simulink model "Current_Fed_DC_DC_Converter_Code_Equivalent_v4"  (R2020a)
settings: Solver=ode3  StartTime=0.0  StopTime=0.4  MaxStep=1e-5  MinStep=1e-7  RelTol=1e-6
InitFcn:
  | %Supply
  | V_supply = 415;
  | f_supply = 50;
  | 
  | %DC_Bus
  | C_filt = 220e-6
  | L_dc = 100e-6;
  | C_out = 560e-3;
  | 
  | %Transformer
  | P_TX = 10e3;
  | V_pri = 36;
  | V_sec = 1;
  | L_leak = 0;
  | R_leak = 0;
  | L_mag = inf;
  | R_mag = inf;
  | 
  | %Control
  | f_sw = 15e3;
  | tss_conv = 0.1;
  | V_ref = 1480;
  | Kp_V = 1;
  | Ki_V = 0.001;
  | I_ref = 2920;
  | Kp_I = 0.025;
  | Ki_I = 0.000001;
  | PS_max = 180;
  | Carr_offset = 1;
  | Carr_scale = 0.5;
  | Duty_scale = 0.01;
  | Duty_fix = 50;
  | Duty_max = 75;
  | Duty_min = 0;
  | f_chop = 1e3;
  | Duty_chop = 40;
  | 
  | %Harmonic_Correction
  | P_inj = 50;
  | f_inj = 50;
  | L_inj = 10e-6;
  | R_inj = 1;
  | Vpri_inj = 1;
  | Vsec_inj = 70;
  | Rleak_inj = 1e-3;
  | Lleak_inj = 12e-6;
  | R_inj = 0.1;
  | Rmag_inj = 1e-3;
  | Lmag_inj = 1e-3;
  | 
  | %Sensor
  | ADC_Res = 4096;
  | I_sense = 1/700;
  | V_sense = 1/50;
  | 
  | %Faults
  | OV_limit = 18.25;
  | UV_limit = 17.5;
  | OC_limit = 515;
  | UC_limit = 22;
  | 
  | %Load
  | R_load = 0.036;
libraries: powerlib x109, powerlib_meascontrol x30, simulink x5, slctrlblks x2
(part 1 of 3)
settings Model: Creator=Duke  LastModifiedBy=Testinglaptop2
settings DataIOCC: ReturnWorkspaceOutputs=off

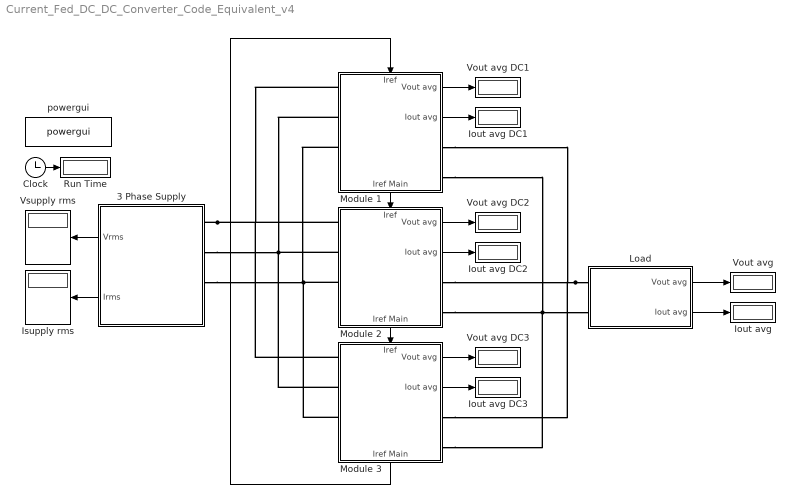
== system Current_Fed_DC_DC_Converter_Code_Equivalent_v4 ==
  3 Phase Supply : Subsystem
      settings: PortSchema="{\"entries\":[{\"content\":{\"sides\":[{\"content\":{\"connectorIds\":[\"Out1\",\"Out2\"]},\"type\":\"ConnectorPlacement.EquallySpacedRectSide\",\"uuid\":\"0ec2aa27-c625-4e75-9974-9a1c04d8f7d1\"},{\"content\":{\"connectorIds\":[\"RConn1\",\"RConn2\",\"RConn3\",\"RConn4\"],\"side\":\"RIGHT\"},\"type\":\"ConnectorPlacement.EquallySpacedRectSide\",\"uuid\":\"47308d37-cd5f-48af-b8fb-0231d0d207f3\"},{\"content\":{\"connectorIds\":[],\"side\":\"TOP\"},\"type\":\"ConnectorPlacement.EquallySpacedRectSide\",\"uuid\":\"36312fad-683d-4b15-bbb8-6a51adddf298\"},{\"content\":{\"connectorIds\":[],\"side\":\"BOTTOM\"},\"type\":\"ConnectorPlacement.EquallySpacedRectSide\",\"uuid\":\"2222870e-1ee8-49e9-8ac2-78ebac8795b0\"}]},\"type\":\"ConnectorPlacement.EquallySpacedConnector\",\"uuid\":\"d2540331-bb7c-4989-bdfb-e9d86418b7e1\"}],\"packageUris\":[\"http://schema.mathworks.com/mf0/Connector/19700101\"],\"version\":\"1.0\"}"
  Clock : Clock
  Iout avg : Display
  Iout avg DC1 : Display
  Iout avg DC2 : Display
  Iout avg DC3 : Display
  Isupply rms : Display
  Load : Subsystem
  Module 1 : Subsystem
      settings: PortSchema="{\"entries\":[{\"content\":{\"sides\":[{\"content\":{\"connectorIds\":[\"LConn1\",\"LConn2\",\"LConn3\",\"LConn4\"]},\"type\":\"ConnectorPlacement.EquallySpacedRectSide\",\"uuid\":\"6cae0e2c-353b-4935-ad30-0e7f8192a6e9\"},{\"content\":{\"connectorIds\":[\"Out1\",\"Out2\",\"RConn1\",\"RConn2\"],\"side\":\"RIGHT\"},\"type\":\"ConnectorPlacement.EquallySpacedRectSide\",\"uuid\":\"f189d0b5-f9e6-4211-8a45-ed2746b7bcfd\"},{\"content\":{\"connectorIds\":[\"In1\"],\"side\":\"TOP\"},\"type\":\"ConnectorPlacement.EquallySpacedRectSide\",\"uuid\":\"18788e66-a885-4273-91b7-13b54a877d5d\"},{\"content\":{\"connectorIds\":[\"Out3\"],\"side\":\"BOTTOM\"},\"type\":\"ConnectorPlacement.EquallySpacedRectSide\",\"uuid\":\"bb6cd510-79be-413f-a402-cf5e288de2de\"}]},\"type\":\"ConnectorPlacement.EquallySpacedConnector\",\"uuid\":\"96fd3dee-bad9-4110-8bef-6c3594df368f\"}],\"packageUris\":[\"http://schema.mathworks.com/mf0/Connector/19700101\"],\"version\":\"1.0\"}"
  Module 2 : Subsystem
      settings: PortSchema="{\"entries\":[{\"content\":{\"sides\":[{\"content\":{\"connectorIds\":[\"LConn1\",\"LConn2\",\"LConn3\",\"LConn4\"]},\"type\":\"ConnectorPlacement.EquallySpacedRectSide\",\"uuid\":\"6cae0e2c-353b-4935-ad30-0e7f8192a6e9\"},{\"content\":{\"connectorIds\":[\"Out1\",\"Out2\",\"RConn1\",\"RConn2\"],\"side\":\"RIGHT\"},\"type\":\"ConnectorPlacement.EquallySpacedRectSide\",\"uuid\":\"f189d0b5-f9e6-4211-8a45-ed2746b7bcfd\"},{\"content\":{\"connectorIds\":[\"In1\"],\"side\":\"TOP\"},\"type\":\"ConnectorPlacement.EquallySpacedRectSide\",\"uuid\":\"18788e66-a885-4273-91b7-13b54a877d5d\"},{\"content\":{\"connectorIds\":[\"Out3\"],\"side\":\"BOTTOM\"},\"type\":\"ConnectorPlacement.EquallySpacedRectSide\",\"uuid\":\"bb6cd510-79be-413f-a402-cf5e288de2de\"}]},\"type\":\"ConnectorPlacement.EquallySpacedConnector\",\"uuid\":\"96fd3dee-bad9-4110-8bef-6c3594df368f\"}],\"packageUris\":[\"http://schema.mathworks.com/mf0/Connector/19700101\"],\"version\":\"1.0\"}"
  Module 3 : Subsystem
      settings: PortSchema="{\"entries\":[{\"content\":{\"sides\":[{\"content\":{\"connectorIds\":[\"LConn1\",\"LConn2\",\"LConn3\",\"LConn4\"]},\"type\":\"ConnectorPlacement.EquallySpacedRectSide\",\"uuid\":\"6cae0e2c-353b-4935-ad30-0e7f8192a6e9\"},{\"content\":{\"connectorIds\":[\"Out1\",\"Out2\",\"RConn1\",\"RConn2\"],\"side\":\"RIGHT\"},\"type\":\"ConnectorPlacement.EquallySpacedRectSide\",\"uuid\":\"f189d0b5-f9e6-4211-8a45-ed2746b7bcfd\"},{\"content\":{\"connectorIds\":[\"In1\"],\"side\":\"TOP\"},\"type\":\"ConnectorPlacement.EquallySpacedRectSide\",\"uuid\":\"18788e66-a885-4273-91b7-13b54a877d5d\"},{\"content\":{\"connectorIds\":[\"Out3\"],\"side\":\"BOTTOM\"},\"type\":\"ConnectorPlacement.EquallySpacedRectSide\",\"uuid\":\"bb6cd510-79be-413f-a402-cf5e288de2de\"}]},\"type\":\"ConnectorPlacement.EquallySpacedConnector\",\"uuid\":\"96fd3dee-bad9-4110-8bef-6c3594df368f\"}],\"packageUris\":[\"http://schema.mathworks.com/mf0/Connector/19700101\"],\"version\":\"1.0\"}"
  Run Time : Display
  Vout avg : Display
  Vout avg DC1 : Display
  Vout avg DC2 : Display
  Vout avg DC3 : Display
  Vsupply rms : Display
  powergui : powerlib/powergui  Priority=1  SimulationMode=Discrete  SampleTime=1e-6  frequency=60  Iterations=50  frequencyindice=0  Pbase=100e6  ErrMax=1e-4  UnitsV=kV  UnitsW=MW  buscounter=0  FunctionMessages=off  echomessages=off  EnableUseOfTLC=off  CurrentSourceSwitches=off  DisableSnubberDevices=off  DisableRonSwitches=off  DisableVfSwitches=off  DisplayEquations=off  AutomaticDiscreteSolvers=off  SolverType=Tustin/Backward Euler (TBE)  Interpol=off  ExternalGateDelay=off  methode=off  Ts=100  x0status=blocks  SPID=on  SwTol=0  HookPort=off  NonlinearTolerance=1e-4  nMaxIteration=100  ContinueOnMaxIteration=off  RestoreLinks=warning  ResistiveCurrentMeasurement=off  Frange=[0:2:500]  Ylog=off  Xlog=on  ShowGrid=off  save=off  variable=ZData  structure=Supply  ZoomFFT=off  StartTime=0.1  cycles=5  DisplayStyle=1  fundamental=50  FreqAxis=off  MaxFrequency=1000  frequencyindicesteady=1  RmsSteady=1  display=off
  wires:
  Clock/1 -> Run Time/1
  Load/2(Iout avg) -> Iout avg/1
  Load/1(Vout avg) -> Vout avg/1
  Module 1/1(Vout avg) -> Vout avg DC1/1
  Module 1/2(Iout avg) -> Iout avg DC1/1
  3 Phase Supply/2(Irms) -> Isupply rms/1
  3 Phase Supply/1(Vrms) -> Vsupply rms/1
  Module 2/2(Iout avg) -> Iout avg DC2/1
  Module 2/1(Vout avg) -> Vout avg DC2/1
  Module 1/3(Iref Main) -> Module 2/1(Iref)
  Module 2/3(Iref Main) -> Module 3/1(Iref)
  Module 3/3(Iref Main) -> Module 1/1(Iref)
  Module 3/1(Vout avg) -> Vout avg DC3/1
  Module 3/2(Iout avg) -> Iout avg DC3/1
  connections:
  3 Phase Supply/RConn1 -- Module 3/LConn1 -- Module 1/LConn1 -- Module 2/LConn1
  Module 1/LConn3 -- 3 Phase Supply/RConn3 -- Module 3/LConn3 -- Module 2/LConn3
  Module 2/RConn2 -- Load/LConn2 -- Module 3/RConn2 -- Module 1/RConn2
  Load/LConn1 -- Module 3/RConn1 -- Module 1/RConn1 -- Module 2/RConn1
  3 Phase Supply/RConn2 -- Module 3/LConn2 -- Module 1/LConn2 -- Module 2/LConn2

== system Current_Fed_DC_DC_Converter_Code_Equivalent_v4/3 Phase Supply ==
  3 Phase Source : powerlib/Electrical Sources/Three-Phase Programmable Voltage Source  PositiveSequence="[V_supply  0 f_supply]"  VariationEntity=None  VariationType=Table of time-amplitude pairs  VariationTypeAlt=Step  VariationStep=0.5  VariationRate=10  VariationMagnitude=0.3  VariationFrequency=2  VariationTiming=[1 2]  VariationPhaseA=off  Amplitudes=[1 0.8 1.2 1.0]  TimeValues=[0 0.1 0.15 0.2]  HarmonicGeneration=off  HarmonicA=[3 0.2 -25 0]  HarmonicB=[2 0.15 35 2]  Timing="[0.05  3]"  BusType=swing  Pref=0  Qref=0  Qmin=-inf  Qmax=inf
  Measurement Input : Subsystem
      settings: PortSchema="{\"entries\":[{\"content\":{\"sides\":[{\"content\":{\"connectorIds\":[\"LConn1\",\"LConn2\",\"LConn3\"]},\"type\":\"ConnectorPlacement.EquallySpacedRectSide\",\"uuid\":\"3be9e5d9-1b35-404b-9f43-9e3a478b191c\"},{\"content\":{\"connectorIds\":[\"RConn1\",\"RConn2\",\"RConn3\"],\"side\":\"RIGHT\"},\"type\":\"ConnectorPlacement.EquallySpacedRectSide\",\"uuid\":\"eba31e05-cbe5-4e3c-a514-94f682603724\"},{\"content\":{\"connectorIds\":[],\"side\":\"TOP\"},\"type\":\"ConnectorPlacement.EquallySpacedRectSide\",\"uuid\":\"b07c13d9-dc8e-463c-8536-a0457c056d42\"},{\"content\":{\"connectorIds\":[\"Out1\",\"Out2\"],\"side\":\"BOTTOM\"},\"type\":\"ConnectorPlacement.EquallySpacedRectSide\",\"uuid\":\"1df26e5f-c204-4844-b869-5c4c651719e7\"}]},\"type\":\"ConnectorPlacement.EquallySpacedConnector\",\"uuid\":\"ca8d1314-165f-4aba-a39c-e8b968dfc3e9\"}],\"packageUris\":[\"http://schema.mathworks.com/mf0/Connector/19700101\"],\"version\":\"1.0\"}"
  Rphase : PMIOPort  Side=Right
  Yphase : PMIOPort  Port=2  Side=Right
  Bphase : PMIOPort  Port=3  Side=Right
  Neutral : PMIOPort  Port=4  Side=Right
  Vrms : Outport
  Irms : Outport  Port=2
  wires:
  Measurement Input/2(Vrms) -> Vrms/1
  Measurement Input/1(Irms) -> Irms/1
  connections:
  Measurement Input/RConn1 -- Rphase/RConn1
  Measurement Input/RConn2 -- Yphase/RConn1
  3 Phase Source/LConn1 -- Neutral/RConn1
  Measurement Input/RConn3 -- Bphase/RConn1
  3 Phase Source/RConn2 -- Measurement Input/LConn2
  3 Phase Source/RConn1 -- Measurement Input/LConn1
  3 Phase Source/RConn3 -- Measurement Input/LConn3

== system Current_Fed_DC_DC_Converter_Code_Equivalent_v4/Load ==
  Io avg : powerlib_meascontrol/Measurements/Mean  Freq=f_supply  Vinit=0  Ts=0
  Iout : powerlib/Measurements/Current Measurement  PhasorSimulation=off  OutputType=Complex  PSBequivalent=0
  Load 1 : powerlib/Elements/Series RLC Branch  LConnTagsString=__new0  RConnTagsString=__new0  BranchType=R  Resistance=R_load  Inductance=1e-3  SetiL0=off  InitialCurrent=0  Capacitance=1e-6  Setx0=off  InitialVoltage=0  Measurements=None
  Load 2 : powerlib/Elements/Series RLC Branch  LConnTagsString=__new0  RConnTagsString=__new0  BranchType=R  Resistance=R_load  Inductance=1e-3  SetiL0=off  InitialCurrent=0  Capacitance=1e-6  Setx0=off  InitialVoltage=0  Measurements=None
  Load 3 : powerlib/Elements/Series RLC Branch  LConnTagsString=__new0  RConnTagsString=__new0  BranchType=R  Resistance=R_load  Inductance=1e-3  SetiL0=off  InitialCurrent=0  Capacitance=1e-6  Setx0=off  InitialVoltage=0  Measurements=None
  Output Parameters : Scope  NumInputPorts=2
  Vo avg : powerlib_meascontrol/Measurements/Mean  Freq=f_supply  Vinit=0  Ts=0
  Vout : powerlib/Measurements/Voltage Measurement  PhasorSimulation=off  OutputType=Complex  PSBequivalent=0
  +ve : PMIOPort  Side=Left
  -ve : PMIOPort  Port=2  Side=Left
  Vout avg : Outport
  Iout avg : Outport  Port=2
  wires:
  Io avg/1 -> Iout avg/1  "Io avg"
  Vo avg/1 -> Vout avg/1  "Vo avg"
  Iout/1 -> Io avg/1, Output Parameters/1  "Iout"
  Vout/1 -> Vo avg/1, Output Parameters/2  "Vout"
  connections:
  Vout/LConn2 -- -ve/RConn1 -- Load 1/RConn1 -- Load 2/RConn1 -- Load 3/RConn1
  Iout/LConn1 -- +ve/RConn1
  Vout/LConn1 -- Load 2/LConn1 -- Load 1/LConn1 -- Iout/RConn1 -- Load 3/LConn1

== system Current_Fed_DC_DC_Converter_Code_Equivalent_v4/Module 1 ==
  Iref : Inport
  3 Phase Rectifier : Subsystem
  DC DC Converter : Subsystem
      settings: PortSchema="{\"entries\":[{\"content\":{\"sides\":[{\"content\":{\"connectorIds\":[\"LConn1\",\"LConn2\"]},\"type\":\"ConnectorPlacement.EquallySpacedRectSide\",\"uuid\":\"37f51f67-5e78-4255-afaf-84866755c3fb\"},{\"content\":{\"connectorIds\":[\"RConn1\",\"RConn2\"],\"side\":\"RIGHT\"},\"type\":\"ConnectorPlacement.EquallySpacedRectSide\",\"uuid\":\"2b53282d-d294-4b9e-9ae3-da15b818eb82\"},{\"content\":{\"connectorIds\":[\"In1\"],\"side\":\"TOP\"},\"type\":\"ConnectorPlacement.EquallySpacedRectSide\",\"uuid\":\"215168e2-cc4d-42b6-b915-d0598b09a452\"},{\"content\":{\"connectorIds\":[\"Out1\",\"Out2\",\"Out3\"],\"side\":\"BOTTOM\"},\"type\":\"ConnectorPlacement.EquallySpacedRectSide\",\"uuid\":\"f9f369b9-2556-4108-8119-ee65139e69f0\"}]},\"type\":\"ConnectorPlacement.EquallySpacedConnector\",\"uuid\":\"d8162db6-aadc-4169-8971-befd1c7fce06\"}],\"packageUris\":[\"http://schema.mathworks.com/mf0/Connector/19700101\"],\"version\":\"1.0\"}"
  Rphase : PMIOPort  Side=Left
  Yphase : PMIOPort  Port=2  Side=Left
  Bphase : PMIOPort  Port=3  Side=Left
  +ve OUT : PMIOPort  Port=4  Side=Right
  -ve OUT : PMIOPort  Port=5  Side=Right
  Neutral : PMIOPort  Port=6  Side=Left
  Vout avg : Outport
  Iout avg : Outport  Port=2
  Iref Main : Outport  Port=3
  wires:
  DC DC Converter/3(Vdc avg) -> Vout avg/1
  DC DC Converter/2(Idc avg) -> Iout avg/1
  DC DC Converter/1(Iref Main) -> Iref Main/1
  Iref/1 -> DC DC Converter/1(Iref)
  connections:
  3 Phase Rectifier/LConn3 -- Bphase/RConn1
  DC DC Converter/LConn1 -- 3 Phase Rectifier/RConn1
  DC DC Converter/LConn2 -- 3 Phase Rectifier/RConn2
  DC DC Converter/RConn2 -- -ve OUT/RConn1
  DC DC Converter/RConn1 -- +ve OUT/RConn1
  3 Phase Rectifier/LConn2 -- Yphase/RConn1
  3 Phase Rectifier/LConn1 -- Rphase/RConn1
  Neutral/RConn1 -- 3 Phase Rectifier/LConn4

== system Current_Fed_DC_DC_Converter_Code_Equivalent_v4/Module 2 ==
  Iref : Inport
  3 Phase Rectifier : Subsystem
  DC DC Converter : Subsystem
      settings: PortSchema="{\"entries\":[{\"content\":{\"sides\":[{\"content\":{\"connectorIds\":[\"LConn1\",\"LConn2\"]},\"type\":\"ConnectorPlacement.EquallySpacedRectSide\",\"uuid\":\"37f51f67-5e78-4255-afaf-84866755c3fb\"},{\"content\":{\"connectorIds\":[\"RConn1\",\"RConn2\"],\"side\":\"RIGHT\"},\"type\":\"ConnectorPlacement.EquallySpacedRectSide\",\"uuid\":\"2b53282d-d294-4b9e-9ae3-da15b818eb82\"},{\"content\":{\"connectorIds\":[\"In1\"],\"side\":\"TOP\"},\"type\":\"ConnectorPlacement.EquallySpacedRectSide\",\"uuid\":\"215168e2-cc4d-42b6-b915-d0598b09a452\"},{\"content\":{\"connectorIds\":[\"Out1\",\"Out2\",\"Out3\"],\"side\":\"BOTTOM\"},\"type\":\"ConnectorPlacement.EquallySpacedRectSide\",\"uuid\":\"f9f369b9-2556-4108-8119-ee65139e69f0\"}]},\"type\":\"ConnectorPlacement.EquallySpacedConnector\",\"uuid\":\"d8162db6-aadc-4169-8971-befd1c7fce06\"}],\"packageUris\":[\"http://schema.mathworks.com/mf0/Connector/19700101\"],\"version\":\"1.0\"}"
  Rphase : PMIOPort  Side=Left
  Yphase : PMIOPort  Port=2  Side=Left
  Bphase : PMIOPort  Port=3  Side=Left
  +ve OUT : PMIOPort  Port=4  Side=Right
  -ve OUT : PMIOPort  Port=5  Side=Right
  Neutral : PMIOPort  Port=6  Side=Left
  Vout avg : Outport
  Iout avg : Outport  Port=2
  Iref Main : Outport  Port=3
  wires:
  Iref/1 -> DC DC Converter/1(Iref)
  DC DC Converter/1(Iref Main) -> Iref Main/1
  DC DC Converter/2(Idc avg) -> Iout avg/1
  DC DC Converter/3(Vdc avg) -> Vout avg/1
  connections:
  Neutral/RConn1 -- 3 Phase Rectifier/LConn4
  3 Phase Rectifier/LConn1 -- Rphase/RConn1
  3 Phase Rectifier/LConn2 -- Yphase/RConn1
  DC DC Converter/RConn1 -- +ve OUT/RConn1
  DC DC Converter/RConn2 -- -ve OUT/RConn1
  DC DC Converter/LConn2 -- 3 Phase Rectifier/RConn2
  DC DC Converter/LConn1 -- 3 Phase Rectifier/RConn1
  3 Phase Rectifier/LConn3 -- Bphase/RConn1

== system Current_Fed_DC_DC_Converter_Code_Equivalent_v4/Module 3 ==
  Iref : Inport
  3 Phase Rectifier : Subsystem
  DC DC Converter : Subsystem
      settings: PortSchema="{\"entries\":[{\"content\":{\"sides\":[{\"content\":{\"connectorIds\":[\"LConn1\",\"LConn2\"]},\"type\":\"ConnectorPlacement.EquallySpacedRectSide\",\"uuid\":\"37f51f67-5e78-4255-afaf-84866755c3fb\"},{\"content\":{\"connectorIds\":[\"RConn1\",\"RConn2\"],\"side\":\"RIGHT\"},\"type\":\"ConnectorPlacement.EquallySpacedRectSide\",\"uuid\":\"2b53282d-d294-4b9e-9ae3-da15b818eb82\"},{\"content\":{\"connectorIds\":[\"In1\"],\"side\":\"TOP\"},\"type\":\"ConnectorPlacement.EquallySpacedRectSide\",\"uuid\":\"215168e2-cc4d-42b6-b915-d0598b09a452\"},{\"content\":{\"connectorIds\":[\"Out1\",\"Out2\",\"Out3\"],\"side\":\"BOTTOM\"},\"type\":\"ConnectorPlacement.EquallySpacedRectSide\",\"uuid\":\"f9f369b9-2556-4108-8119-ee65139e69f0\"}]},\"type\":\"ConnectorPlacement.EquallySpacedConnector\",\"uuid\":\"d8162db6-aadc-4169-8971-befd1c7fce06\"}],\"packageUris\":[\"http://schema.mathworks.com/mf0/Connector/19700101\"],\"version\":\"1.0\"}"
  Rphase : PMIOPort  Side=Left
  Yphase : PMIOPort  Port=2  Side=Left
  Bphase : PMIOPort  Port=3  Side=Left
  +ve OUT : PMIOPort  Port=4  Side=Right
  -ve OUT : PMIOPort  Port=5  Side=Right
  Neutral : PMIOPort  Port=6  Side=Left
  Vout avg : Outport
  Iout avg : Outport  Port=2
  Iref Main : Outport  Port=3
  wires:
  Iref/1 -> DC DC Converter/1(Iref)
  DC DC Converter/1(Iref Main) -> Iref Main/1
  DC DC Converter/2(Idc avg) -> Iout avg/1
  DC DC Converter/3(Vdc avg) -> Vout avg/1
  connections:
  Neutral/RConn1 -- 3 Phase Rectifier/LConn4
  3 Phase Rectifier/LConn1 -- Rphase/RConn1
  3 Phase Rectifier/LConn2 -- Yphase/RConn1
  DC DC Converter/RConn1 -- +ve OUT/RConn1
  DC DC Converter/RConn2 -- -ve OUT/RConn1
  DC DC Converter/LConn2 -- 3 Phase Rectifier/RConn2
  DC DC Converter/LConn1 -- 3 Phase Rectifier/RConn1
  3 Phase Rectifier/LConn3 -- Bphase/RConn1

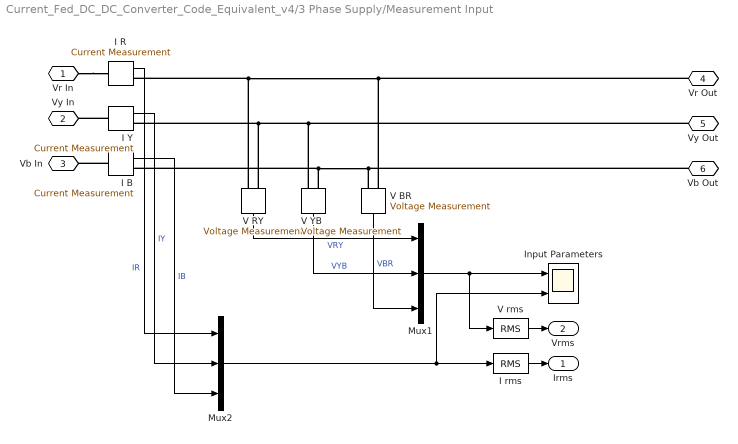
== system Current_Fed_DC_DC_Converter_Code_Equivalent_v4/3 Phase Supply/Measurement Input ==
  I B : powerlib/Measurements/Current Measurement  PhasorSimulation=off  OutputType=Complex  PSBequivalent=0
  I R : powerlib/Measurements/Current Measurement  PhasorSimulation=off  OutputType=Complex  PSBequivalent=0
  I Y : powerlib/Measurements/Current Measurement  PhasorSimulation=off  OutputType=Complex  PSBequivalent=0
  I rms : powerlib_meascontrol/Measurements/RMS  TrueRMS=on  Freq=f_supply  RMSInit=0  Ts=0
  Input Parameters : Scope  NumInputPorts=2
  Mux1 : Mux  Inputs=3
  Mux2 : Mux  Inputs=3
  V BR : powerlib/Measurements/Voltage Measurement  PhasorSimulation=off  OutputType=Complex  PSBequivalent=0
  V RY : powerlib/Measurements/Voltage Measurement  PhasorSimulation=off  OutputType=Complex  PSBequivalent=0
  V YB : powerlib/Measurements/Voltage Measurement  PhasorSimulation=off  OutputType=Complex  PSBequivalent=0
  V rms : powerlib_meascontrol/Measurements/RMS  TrueRMS=on  Freq=f_supply  RMSInit=0  Ts=0
  Vr In : PMIOPort  Side=Left
  Vy In : PMIOPort  Port=2  Side=Left
  Vb In : PMIOPort  Port=3  Side=Left
  Vr Out : PMIOPort  Port=4  Side=Right
  Vy Out : PMIOPort  Port=5  Side=Right
  Vb Out : PMIOPort  Port=6  Side=Right
  Irms : Outport
  Vrms : Outport  Port=2
  wires:
  Mux2/1 -> Input Parameters/2, I rms/1
  V RY/1 -> Mux1/1  "VRY"
  Mux1/1 -> Input Parameters/1, V rms/1
  I B/1 -> Mux2/3  "IB"
  I Y/1 -> Mux2/2  "IY"
  I R/1 -> Mux2/1  "IR"
  V BR/1 -> Mux1/3  "VBR"
  V YB/1 -> Mux1/2  "VYB"
  I rms/1 -> Irms/1
  V rms/1 -> Vrms/1
  connections:
  V YB/LConn2 -- I B/RConn1 -- Vb Out/RConn1 -- V BR/LConn1
  V RY/LConn1 -- Vr Out/RConn1 -- V BR/LConn2 -- I R/RConn1
  Vr In/RConn1 -- I R/LConn1
  V RY/LConn2 -- Vy Out/RConn1 -- V YB/LConn1 -- I Y/RConn1
  I B/LConn1 -- Vb In/RConn1
  I Y/LConn1 -- Vy In/RConn1

== system Current_Fed_DC_DC_Converter_Code_Equivalent_v4/Module 1/3 Phase Rectifier ==
  3 Phase Rectifier : Subsystem
  Filter : Subsystem
  Rphase : PMIOPort  Side=Left
  Yphase : PMIOPort  Port=2  Side=Left
  Bphase : PMIOPort  Port=3  Side=Left
  +ve : PMIOPort  Port=4  Side=Right
  -ve : PMIOPort  Port=5  Side=Right
  Neutral : PMIOPort  Port=6  Side=Left
  connections:
  Bphase/RConn1 -- 3 Phase Rectifier/LConn3
  Yphase/RConn1 -- 3 Phase Rectifier/LConn2
  3 Phase Rectifier/LConn1 -- Rphase/RConn1
  -ve/RConn1 -- Filter/RConn3
  3 Phase Rectifier/RConn1 -- Filter/LConn1
  +ve/RConn1 -- Filter/RConn1
  3 Phase Rectifier/RConn2 -- Filter/LConn2
  Neutral/RConn1 -- Filter/RConn2

== system Current_Fed_DC_DC_Converter_Code_Equivalent_v4/Module 1/DC DC Converter ==
  Iref : Inport
  Centre Tap Rectifier : Subsystem
  Chopper : Subsystem
      settings: PortSchema="{\"entries\":[{\"content\":{\"sides\":[{\"content\":{\"connectorIds\":[\"LConn1\",\"LConn2\"]},\"type\":\"ConnectorPlacement.EquallySpacedRectSide\",\"uuid\":\"27b0ffc8-d442-4d0b-b35b-d90ae246715a\"},{\"content\":{\"connectorIds\":[\"RConn1\",\"RConn2\"],\"side\":\"RIGHT\"},\"type\":\"ConnectorPlacement.EquallySpacedRectSide\",\"uuid\":\"032ddb76-2114-4733-a261-6d5dce4f9c1e\"},{\"content\":{\"connectorIds\":[\"Out3\",\"Out4\"],\"side\":\"TOP\"},\"type\":\"ConnectorPlacement.EquallySpacedRectSide\",\"uuid\":\"ba624cc1-6780-4a11-b503-2af71fb179ff\"},{\"content\":{\"connectorIds\":[\"Out1\",\"Out2\"],\"side\":\"BOTTOM\"},\"type\":\"ConnectorPlacement.EquallySpacedRectSide\",\"uuid\":\"1ef588f8-a75b-4578-aeed-4d7f75c968c1\"}]},\"type\":\"ConnectorPlacement.EquallySpacedConnector\",\"uuid\":\"9ac1a3f6-3708-41de-9f61-69d76e8a5f0b\"}],\"packageUris\":[\"http://schema.mathworks.com/mf0/Connector/19700101\"],\"version\":\"1.0\"}"
  DC Bus : Subsystem
  Filter : Subsystem
  HF Transformer : Subsystem
  Inverter : Subsystem
      settings: PortSchema="{\"entries\":[{\"content\":{\"sides\":[{\"content\":{\"connectorIds\":[\"LConn1\",\"LConn2\"]},\"type\":\"ConnectorPlacement.EquallySpacedRectSide\",\"uuid\":\"f6e7bef4-cb5f-453b-95e0-57d178fdcdab\"},{\"content\":{\"connectorIds\":[\"RConn1\",\"RConn2\"],\"side\":\"RIGHT\"},\"type\":\"ConnectorPlacement.EquallySpacedRectSide\",\"uuid\":\"145c04da-1f90-4c9a-a0a3-45235f26f3c1\"},{\"content\":{\"connectorIds\":[\"In1\",\"In2\",\"In3\"],\"side\":\"TOP\"},\"type\":\"ConnectorPlacement.EquallySpacedRectSide\",\"uuid\":\"e53d65e9-ce43-4967-b260-28202a06c4d8\"},{\"content\":{\"connectorIds\":[\"Out1\"],\"side\":\"BOTTOM\"},\"type\":\"ConnectorPlacement.EquallySpacedRectSide\",\"uuid\":\"b31c56a6-13fe-4b55-8dac-b140b94eae9e\"}]},\"type\":\"ConnectorPlacement.EquallySpacedConnector\",\"uuid\":\"a4a232a8-d845-4efa-a1c4-da2bb120aefc\"}],\"packageUris\":[\"http://schema.mathworks.com/mf0/Connector/19700101\"],\"version\":\"1.0\"}"
  Sensor : Subsystem
  +ve IN : PMIOPort  Side=Left
  -ve IN : PMIOPort  Port=2  Side=Left
  +ve OUT : PMIOPort  Port=3  Side=Right
  -ve OUT : PMIOPort  Port=4  Side=Right
  Iref Main : Outport
  Idc avg : Outport  Port=2
  Vdc avg : Outport  Port=3
  wires:
  Inverter/1(Iref Main) -> Iref Main/1
  Iref/1 -> Inverter/1(Iref)
  Chopper/2(Vdc avg) -> Vdc avg/1
  Chopper/1(Idc avg) -> Idc avg/1
  Chopper/3(Vdc) -> Sensor/2(Vin)
  Chopper/4(" Idc") -> Sensor/1(Iin)
  Sensor/2(Vout) -> Inverter/3(Vfeed)
  Sensor/1(Iout) -> Inverter/2(Ifeed)
  connections:
  DC Bus/LConn2 -- -ve IN/RConn1
  DC Bus/LConn1 -- +ve IN/RConn1
  DC Bus/RConn1 -- Inverter/LConn1
  DC Bus/RConn2 -- Inverter/LConn2
  Filter/LConn2 -- Centre Tap Rectifier/RConn2
  Filter/LConn1 -- Centre Tap Rectifier/RConn1
  HF Transformer/RConn3 -- Centre Tap Rectifier/LConn3
  HF Transformer/RConn1 -- Centre Tap Rectifier/LConn1
  HF Transformer/LConn2 -- Inverter/RConn2
  HF Transformer/LConn1 -- Inverter/RConn1
  HF Transformer/RConn2 -- Centre Tap Rectifier/LConn2
  Chopper/LConn1 -- Filter/RConn1
  +ve OUT/RConn1 -- Chopper/RConn1
  Chopper/LConn2 -- Filter/RConn2
  -ve OUT/RConn1 -- Chopper/RConn2

== system Current_Fed_DC_DC_Converter_Code_Equivalent_v4/Module 2/3 Phase Rectifier ==
  3 Phase Rectifier : Subsystem
  Filter : Subsystem
  Rphase : PMIOPort  Side=Left
  Yphase : PMIOPort  Port=2  Side=Left
  Bphase : PMIOPort  Port=3  Side=Left
  +ve : PMIOPort  Port=4  Side=Right
  -ve : PMIOPort  Port=5  Side=Right
  Neutral : PMIOPort  Port=6  Side=Left
  connections:
  Neutral/RConn1 -- Filter/RConn2
  3 Phase Rectifier/RConn2 -- Filter/LConn2
  +ve/RConn1 -- Filter/RConn1
  3 Phase Rectifier/RConn1 -- Filter/LConn1
  -ve/RConn1 -- Filter/RConn3
  3 Phase Rectifier/LConn1 -- Rphase/RConn1
  Yphase/RConn1 -- 3 Phase Rectifier/LConn2
  Bphase/RConn1 -- 3 Phase Rectifier/LConn3

== system Current_Fed_DC_DC_Converter_Code_Equivalent_v4/Module 2/DC DC Converter ==
  Iref : Inport
  Centre Tap Rectifier : Subsystem
  Chopper : Subsystem
      settings: PortSchema="{\"entries\":[{\"content\":{\"sides\":[{\"content\":{\"connectorIds\":[\"LConn1\",\"LConn2\"]},\"type\":\"ConnectorPlacement.EquallySpacedRectSide\",\"uuid\":\"27b0ffc8-d442-4d0b-b35b-d90ae246715a\"},{\"content\":{\"connectorIds\":[\"RConn1\",\"RConn2\"],\"side\":\"RIGHT\"},\"type\":\"ConnectorPlacement.EquallySpacedRectSide\",\"uuid\":\"032ddb76-2114-4733-a261-6d5dce4f9c1e\"},{\"content\":{\"connectorIds\":[\"Out3\",\"Out4\"],\"side\":\"TOP\"},\"type\":\"ConnectorPlacement.EquallySpacedRectSide\",\"uuid\":\"ba624cc1-6780-4a11-b503-2af71fb179ff\"},{\"content\":{\"connectorIds\":[\"Out1\",\"Out2\"],\"side\":\"BOTTOM\"},\"type\":\"ConnectorPlacement.EquallySpacedRectSide\",\"uuid\":\"1ef588f8-a75b-4578-aeed-4d7f75c968c1\"}]},\"type\":\"ConnectorPlacement.EquallySpacedConnector\",\"uuid\":\"9ac1a3f6-3708-41de-9f61-69d76e8a5f0b\"}],\"packageUris\":[\"http://schema.mathworks.com/mf0/Connector/19700101\"],\"version\":\"1.0\"}"
  DC Bus : Subsystem
  Filter : Subsystem
  HF Transformer : Subsystem
  Inverter : Subsystem
      settings: PortSchema="{\"entries\":[{\"content\":{\"sides\":[{\"content\":{\"connectorIds\":[\"LConn1\",\"LConn2\"]},\"type\":\"ConnectorPlacement.EquallySpacedRectSide\",\"uuid\":\"f6e7bef4-cb5f-453b-95e0-57d178fdcdab\"},{\"content\":{\"connectorIds\":[\"RConn1\",\"RConn2\"],\"side\":\"RIGHT\"},\"type\":\"ConnectorPlacement.EquallySpacedRectSide\",\"uuid\":\"145c04da-1f90-4c9a-a0a3-45235f26f3c1\"},{\"content\":{\"connectorIds\":[\"In1\",\"In2\",\"In3\"],\"side\":\"TOP\"},\"type\":\"ConnectorPlacement.EquallySpacedRectSide\",\"uuid\":\"e53d65e9-ce43-4967-b260-28202a06c4d8\"},{\"content\":{\"connectorIds\":[\"Out1\"],\"side\":\"BOTTOM\"},\"type\":\"ConnectorPlacement.EquallySpacedRectSide\",\"uuid\":\"b31c56a6-13fe-4b55-8dac-b140b94eae9e\"}]},\"type\":\"ConnectorPlacement.EquallySpacedConnector\",\"uuid\":\"a4a232a8-d845-4efa-a1c4-da2bb120aefc\"}],\"packageUris\":[\"http://schema.mathworks.com/mf0/Connector/19700101\"],\"version\":\"1.0\"}"
  Sensor : Subsystem
  +ve IN : PMIOPort  Side=Left
  -ve IN : PMIOPort  Port=2  Side=Left
  +ve OUT : PMIOPort  Port=3  Side=Right
  -ve OUT : PMIOPort  Port=4  Side=Right
  Iref Main : Outport
  Idc avg : Outport  Port=2
  Vdc avg : Outport  Port=3
  wires:
  Sensor/2(Vout) -> Inverter/3(Vfeed)
  Sensor/1(Iout) -> Inverter/2(Ifeed)
  Chopper/4(" Idc") -> Sensor/1(Iin)
  Chopper/3(Vdc) -> Sensor/2(Vin)
  Chopper/1(Idc avg) -> Idc avg/1
  Chopper/2(Vdc avg) -> Vdc avg/1
  Iref/1 -> Inverter/1(Iref)
  Inverter/1(Iref Main) -> Iref Main/1
  connections:
  -ve OUT/RConn1 -- Chopper/RConn2
  Chopper/LConn2 -- Filter/RConn2
  +ve OUT/RConn1 -- Chopper/RConn1
  Chopper/LConn1 -- Filter/RConn1
  HF Transformer/RConn2 -- Centre Tap Rectifier/LConn2
  HF Transformer/LConn1 -- Inverter/RConn1
  HF Transformer/LConn2 -- Inverter/RConn2
  HF Transformer/RConn1 -- Centre Tap Rectifier/LConn1
  HF Transformer/RConn3 -- Centre Tap Rectifier/LConn3
  Filter/LConn1 -- Centre Tap Rectifier/RConn1
  Filter/LConn2 -- Centre Tap Rectifier/RConn2
  DC Bus/RConn2 -- Inverter/LConn2
  DC Bus/RConn1 -- Inverter/LConn1
  DC Bus/LConn1 -- +ve IN/RConn1
  DC Bus/LConn2 -- -ve IN/RConn1

== system Current_Fed_DC_DC_Converter_Code_Equivalent_v4/Module 3/3 Phase Rectifier ==
  3 Phase Rectifier : Subsystem
  Filter : Subsystem
  Rphase : PMIOPort  Side=Left
  Yphase : PMIOPort  Port=2  Side=Left
  Bphase : PMIOPort  Port=3  Side=Left
  +ve : PMIOPort  Port=4  Side=Right
  -ve : PMIOPort  Port=5  Side=Right
  Neutral : PMIOPort  Port=6  Side=Left
  connections:
  Neutral/RConn1 -- Filter/RConn2
  3 Phase Rectifier/RConn2 -- Filter/LConn2
  +ve/RConn1 -- Filter/RConn1
  3 Phase Rectifier/RConn1 -- Filter/LConn1
  -ve/RConn1 -- Filter/RConn3
  3 Phase Rectifier/LConn1 -- Rphase/RConn1
  Yphase/RConn1 -- 3 Phase Rectifier/LConn2
  Bphase/RConn1 -- 3 Phase Rectifier/LConn3

== system Current_Fed_DC_DC_Converter_Code_Equivalent_v4/Module 3/DC DC Converter ==
  Iref : Inport
  Centre Tap Rectifier : Subsystem
  Chopper : Subsystem
      settings: PortSchema="{\"entries\":[{\"content\":{\"sides\":[{\"content\":{\"connectorIds\":[\"LConn1\",\"LConn2\"]},\"type\":\"ConnectorPlacement.EquallySpacedRectSide\",\"uuid\":\"27b0ffc8-d442-4d0b-b35b-d90ae246715a\"},{\"content\":{\"connectorIds\":[\"RConn1\",\"RConn2\"],\"side\":\"RIGHT\"},\"type\":\"ConnectorPlacement.EquallySpacedRectSide\",\"uuid\":\"032ddb76-2114-4733-a261-6d5dce4f9c1e\"},{\"content\":{\"connectorIds\":[\"Out3\",\"Out4\"],\"side\":\"TOP\"},\"type\":\"ConnectorPlacement.EquallySpacedRectSide\",\"uuid\":\"ba624cc1-6780-4a11-b503-2af71fb179ff\"},{\"content\":{\"connectorIds\":[\"Out1\",\"Out2\"],\"side\":\"BOTTOM\"},\"type\":\"ConnectorPlacement.EquallySpacedRectSide\",\"uuid\":\"1ef588f8-a75b-4578-aeed-4d7f75c968c1\"}]},\"type\":\"ConnectorPlacement.EquallySpacedConnector\",\"uuid\":\"9ac1a3f6-3708-41de-9f61-69d76e8a5f0b\"}],\"packageUris\":[\"http://schema.mathworks.com/mf0/Connector/19700101\"],\"version\":\"1.0\"}"
  DC Bus : Subsystem
  Filter : Subsystem
  HF Transformer : Subsystem
  Inverter : Subsystem
      settings: PortSchema="{\"entries\":[{\"content\":{\"sides\":[{\"content\":{\"connectorIds\":[\"LConn1\",\"LConn2\"]},\"type\":\"ConnectorPlacement.EquallySpacedRectSide\",\"uuid\":\"f6e7bef4-cb5f-453b-95e0-57d178fdcdab\"},{\"content\":{\"connectorIds\":[\"RConn1\",\"RConn2\"],\"side\":\"RIGHT\"},\"type\":\"ConnectorPlacement.EquallySpacedRectSide\",\"uuid\":\"145c04da-1f90-4c9a-a0a3-45235f26f3c1\"},{\"content\":{\"connectorIds\":[\"In1\",\"In2\",\"In3\"],\"side\":\"TOP\"},\"type\":\"ConnectorPlacement.EquallySpacedRectSide\",\"uuid\":\"e53d65e9-ce43-4967-b260-28202a06c4d8\"},{\"content\":{\"connectorIds\":[\"Out1\"],\"side\":\"BOTTOM\"},\"type\":\"ConnectorPlacement.EquallySpacedRectSide\",\"uuid\":\"b31c56a6-13fe-4b55-8dac-b140b94eae9e\"}]},\"type\":\"ConnectorPlacement.EquallySpacedConnector\",\"uuid\":\"a4a232a8-d845-4efa-a1c4-da2bb120aefc\"}],\"packageUris\":[\"http://schema.mathworks.com/mf0/Connector/19700101\"],\"version\":\"1.0\"}"
  Sensor : Subsystem
  +ve IN : PMIOPort  Side=Left
  -ve IN : PMIOPort  Port=2  Side=Left
  +ve OUT : PMIOPort  Port=3  Side=Right
  -ve OUT : PMIOPort  Port=4  Side=Right
  Iref Main : Outport
  Idc avg : Outport  Port=2
  Vdc avg : Outport  Port=3
  wires:
  Sensor/2(Vout) -> Inverter/3(Vfeed)
  Sensor/1(Iout) -> Inverter/2(Ifeed)
  Chopper/4(" Idc") -> Sensor/1(Iin)
  Chopper/3(Vdc) -> Sensor/2(Vin)
  Chopper/1(Idc avg) -> Idc avg/1
  Chopper/2(Vdc avg) -> Vdc avg/1
  Iref/1 -> Inverter/1(Iref)
  Inverter/1(Iref Main) -> Iref Main/1
  connections:
  -ve OUT/RConn1 -- Chopper/RConn2
  Chopper/LConn2 -- Filter/RConn2
  +ve OUT/RConn1 -- Chopper/RConn1
  Chopper/LConn1 -- Filter/RConn1
  HF Transformer/RConn2 -- Centre Tap Rectifier/LConn2
  HF Transformer/LConn1 -- Inverter/RConn1
  HF Transformer/LConn2 -- Inverter/RConn2
  HF Transformer/RConn1 -- Centre Tap Rectifier/LConn1
  HF Transformer/RConn3 -- Centre Tap Rectifier/LConn3
  Filter/LConn1 -- Centre Tap Rectifier/RConn1
  Filter/LConn2 -- Centre Tap Rectifier/RConn2
  DC Bus/RConn2 -- Inverter/LConn2
  DC Bus/RConn1 -- Inverter/LConn1
  DC Bus/LConn1 -- +ve IN/RConn1
  DC Bus/LConn2 -- -ve IN/RConn1

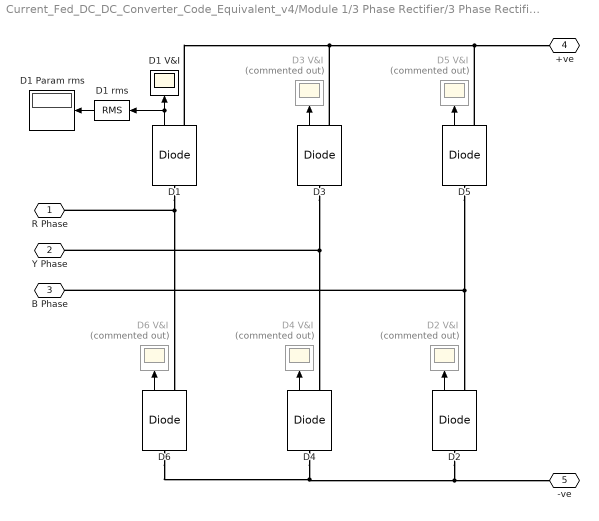
== system Current_Fed_DC_DC_Converter_Code_Equivalent_v4/Module 1/3 Phase Rectifier/3 Phase Rectifier ==
  D{1..6} (6 alike) : powerlib/Power Electronics/Diode  Ron=0.001  Lon=0  Vf=0.8  IC=0  UseSnubber=0  Rs=500  Cs=250e-9  Measurements=on
  D1 V&I : Scope
  D1 Param rms : Display
  D1 rms : powerlib_meascontrol/Measurements/RMS  TrueRMS=on  Freq=f_supply  RMSInit=0  Ts=0
  D2 V&I : Scope  Commented=on
  D3 V&I : Scope  Commented=on
  D4 V&I : Scope  Commented=on
  D5 V&I : Scope  Commented=on
  D6 V&I : Scope  Commented=on
  R Phase : PMIOPort  Side=Left
  Y Phase : PMIOPort  Port=2  Side=Left
  B Phase : PMIOPort  Port=3  Side=Left
  +ve : PMIOPort  Port=4  Side=Right
  -ve : PMIOPort  Port=5  Side=Right
  wires:
  D6/1 -> D6 V&I/1
  D2/1 -> D2 V&I/1
  D5/1 -> D5 V&I/1
  D3/1 -> D3 V&I/1
  D4/1 -> D4 V&I/1
  D1/1 -> D1 rms/1, D1 V&I/1
  D1 rms/1 -> D1 Param rms/1
  connections:
  D1/LConn1 -- D6/RConn1 -- R Phase/RConn1
  D1/RConn1 -- D3/RConn1 -- +ve/RConn1 -- D5/RConn1
  D6/LConn1 -- D4/LConn1 -- D2/LConn1 -- -ve/RConn1
  D3/LConn1 -- D4/RConn1 -- Y Phase/RConn1
  D5/LConn1 -- D2/RConn1 -- B Phase/RConn1

== system Current_Fed_DC_DC_Converter_Code_Equivalent_v4/Module 1/3 Phase Rectifier/Filter ==
  Cdc 1 : powerlib/Elements/Series RLC Branch  LConnTagsString=__new0  RConnTagsString=__new0  BranchType=C  Resistance=1  Inductance=1e-3  SetiL0=off  InitialCurrent=0  Capacitance=2*C_filt  Setx0=off  InitialVoltage=0  Measurements=None
  Cdc 2 : powerlib/Elements/Series RLC Branch  LConnTagsString=__new0  RConnTagsString=__new0  BranchType=C  Resistance=1  Inductance=1e-3  SetiL0=off  InitialCurrent=0  Capacitance=2*C_filt  Setx0=off  InitialVoltage=0  Measurements=None
  DC Bus Filter Parameters : Scope  NumInputPorts=2
  Display : Display
  Display1 : Display
  Io avg : powerlib_meascontrol/Measurements/Mean  Freq=f_supply  Vinit=0  Ts=0
  Iout : powerlib/Measurements/Current Measurement  PhasorSimulation=off  OutputType=Complex  PSBequivalent=0
  Vo avg : powerlib_meascontrol/Measurements/Mean  Freq=f_supply  Vinit=0  Ts=0
  Vout : powerlib/Measurements/Voltage Measurement  PhasorSimulation=off  OutputType=Complex  PSBequivalent=0
  +ve IN : PMIOPort  Side=Left
  -ve In : PMIOPort  Port=2  Side=Left
  +ve OUT : PMIOPort  Port=3  Side=Right
  Mid : PMIOPort  Port=4  Side=Right
  -ve OUT : PMIOPort  Port=5  Side=Right
  wires:
  Iout/1 -> Io avg/1, DC Bus Filter Parameters/1  "Iout"
  Vout/1 -> Vo avg/1, DC Bus Filter Parameters/2  "Vout"
  Io avg/1 -> Display/1  "Io avg"
  Vo avg/1 -> Display1/1  "Vo avg"
  connections:
  Vout/LConn1 -- Cdc 1/LConn1 -- +ve IN/RConn1 -- Iout/LConn1
  Vout/LConn2 -- Cdc 2/RConn1 -- -ve In/RConn1 -- -ve OUT/RConn1
  +ve OUT/RConn1 -- Iout/RConn1
  Cdc 1/RConn1 -- Mid/RConn1 -- Cdc 2/LConn1

== system Current_Fed_DC_DC_Converter_Code_Equivalent_v4/Module 1/DC DC Converter/Centre Tap Rectifier ==
  D Param rms : Display
  D avg : powerlib_meascontrol/Measurements/Mean  Freq=f_supply  Vinit=0  Ts=0
  D1 : powerlib/Power Electronics/Diode  Ron=0.001  Lon=0  Vf=0.8  IC=0  UseSnubber=0  Rs=500  Cs=250e-9  Measurements=on
  D1 V&I : Scope
  D2 : powerlib/Power Electronics/Diode  Ron=0.001  Lon=0  Vf=0.8  IC=0  UseSnubber=0  Rs=500  Cs=250e-9  Measurements=on
  D2 V&I1 : Scope  Commented=on
  Line : PMIOPort  Side=Left
  Centre-tap : PMIOPort  Port=2  Side=Left
  Neutral : PMIOPort  Port=3  Side=Left
  +ve : PMIOPort  Port=4  Side=Right
  -ve : PMIOPort  Port=5  Side=Right
  wires:
  D2/1 -> D2 V&I1/1
  D1/1 -> D avg/1, D1 V&I/1
  D avg/1 -> D Param rms/1
  connections:
  -ve/RConn1 -- Centre-tap/RConn1
  D2/LConn1 -- Neutral/RConn1
  D1/LConn1 -- Line/RConn1
  D2/RConn1 -- +ve/RConn1 -- D1/RConn1

== system Current_Fed_DC_DC_Converter_Code_Equivalent_v4/Module 1/DC DC Converter/Chopper ==
  Chop Pulse Generator : Subsystem
  Fault Detection : Subsystem
  Io avg : powerlib_meascontrol/Measurements/Mean  Freq=f_supply  Vinit=0  Ts=0
  Iout : powerlib/Measurements/Current Measurement  PhasorSimulation=off  OutputType=Complex  PSBequivalent=0
  Out Parameters : Scope  NumInputPorts=2
  Qchop : powerlib/Power Electronics/IGBT  Ron=0.001  Lon=0  Vf=1  Tf=1e-6  Tt=2e-6  IC=0  Rs=1e5  Cs=inf  Measurements=on
  Qchop V&I : Scope  Commented=on
  Rchop : powerlib/Elements/Series RLC Branch  LConnTagsString=__new0  RConnTagsString=__new0  BranchType=R  Resistance=0.1  Inductance=1e-3  SetiL0=off  InitialCurrent=0  Capacitance=1e-6  Setx0=off  InitialVoltage=0  Measurements=None
  Vo avg : powerlib_meascontrol/Measurements/Mean  Freq=f_supply  Vinit=0  Ts=0
  Vout : powerlib/Measurements/Voltage Measurement  PhasorSimulation=off  OutputType=Complex  PSBequivalent=0
  +ve IN : PMIOPort  Side=Left
  -ve IN : PMIOPort  Port=2  Side=Left
  +ve OUT : PMIOPort  Port=3  Side=Right
  -ve OUT : PMIOPort  Port=4  Side=Right
  Idc avg : Outport
  Vdc avg : Outport  Port=2
  Vdc : Outport  Port=3
  " Idc" : Outport  Port=4
  wires:
  Fault Detection/1(OV Fault) -> Chop Pulse Generator/1(Over Voltage Fault)
  Vout/1 -> Fault Detection/1(V Output), Out Parameters/2, Vo avg/1, Vdc/1  "Vout"
  Io avg/1 -> Idc avg/1  "Io avg"
  Iout/1 -> Out Parameters/1, Io avg/1, Fault Detection/2(I Output), " Idc"/1  "Iout"
  Qchop/1 -> Qchop V&I/1
  Vo avg/1 -> Vdc avg/1  "Vo avg"
  Chop Pulse Generator/1(Chop Pulse) -> Qchop/1
  connections:
  Vout/LConn2 -- Rchop/RConn1 -- -ve IN/RConn1 -- -ve OUT/RConn1
  Qchop/LConn1 -- +ve IN/RConn1 -- Iout/LConn1
  Rchop/LConn1 -- Qchop/RConn1
  Vout/LConn1 -- Iout/RConn1 -- +ve OUT/RConn1

== system Current_Fed_DC_DC_Converter_Code_Equivalent_v4/Module 1/DC DC Converter/DC Bus ==
  DC Bus Parameter : Scope  NumInputPorts=2
  Display : Display
  Display1 : Display
  Idc filt : powerlib/Measurements/Current Measurement  PhasorSimulation=off  OutputType=Complex  PSBequivalent=0
  Io avg : powerlib_meascontrol/Measurements/Mean  Freq=f_supply  Vinit=0  Ts=0
  L bus : powerlib/Elements/Series RLC Branch  LConnTagsString=__new0  RConnTagsString=__new0  BranchType=L  Resistance=1  Inductance=L_dc  SetiL0=off  InitialCurrent=0  Capacitance=1e-6  Setx0=off  InitialVoltage=0  Measurements=None
  Vdc : powerlib/Measurements/Voltage Measurement  PhasorSimulation=off  OutputType=Complex  PSBequivalent=0
  Vo avg : powerlib_meascontrol/Measurements/Mean  Freq=f_supply  Vinit=0  Ts=0
  +ve IN : PMIOPort  Side=Left
  -ve IN : PMIOPort  Port=2  Side=Left
  +ve OUT : PMIOPort  Port=3  Side=Right
  -ve OUT : PMIOPort  Port=4  Side=Right
  wires:
  Idc filt/1 -> Io avg/1, DC Bus Parameter/1  "Ifilt"
  Vdc/1 -> Vo avg/1, DC Bus Parameter/2  "Vdc"
  Vo avg/1 -> Display1/1  "Vo avg"
  Io avg/1 -> Display/1  "Io avg"
  connections:
  +ve IN/RConn1 -- L bus/LConn1
  -ve OUT/RConn1 -- -ve IN/RConn1 -- Vdc/LConn2
  L bus/RConn1 -- Vdc/LConn1 -- Idc filt/LConn1
  Idc filt/RConn1 -- +ve OUT/RConn1

== system Current_Fed_DC_DC_Converter_Code_Equivalent_v4/Module 1/DC DC Converter/Filter ==
  C out : powerlib/Elements/Series RLC Branch  LConnTagsString=__new0  RConnTagsString=__new0  BranchType=C  Resistance=10  Inductance=1e-3  SetiL0=off  InitialCurrent=0  Capacitance=C_out  Setx0=off  InitialVoltage=0  Measurements=None
  Display : Display
  Display1 : Display
  I C Filter : powerlib/Measurements/Current Measurement  PhasorSimulation=off  OutputType=Complex  PSBequivalent=0
  I out : powerlib/Measurements/Current Measurement  PhasorSimulation=off  OutputType=Complex  PSBequivalent=0
  Io avg : powerlib_meascontrol/Measurements/Mean  Freq=f_supply  Vinit=0  Ts=0
  Output Filter Parameters : Scope  NumInputPorts=2
  Vo avg : powerlib_meascontrol/Measurements/Mean  Freq=f_supply  Vinit=0  Ts=0
  +ve IN : PMIOPort  Side=Left
  -ve IN : PMIOPort  Port=2  Side=Left
  +ve OUT : PMIOPort  Port=3  Side=Right
  -ve OUT : PMIOPort  Port=4  Side=Right
  wires:
  I out/1 -> Vo avg/1, Output Filter Parameters/1
  I C Filter/1 -> Output Filter Parameters/2, Io avg/1
  Io avg/1 -> Display1/1
  Vo avg/1 -> Display/1
  connections:
  -ve IN/RConn1 -- -ve OUT/RConn1 -- C out/RConn1
  I out/LConn1 -- +ve IN/RConn1 -- I C Filter/LConn1
  I C Filter/RConn1 -- C out/LConn1
  +ve OUT/RConn1 -- I out/RConn1

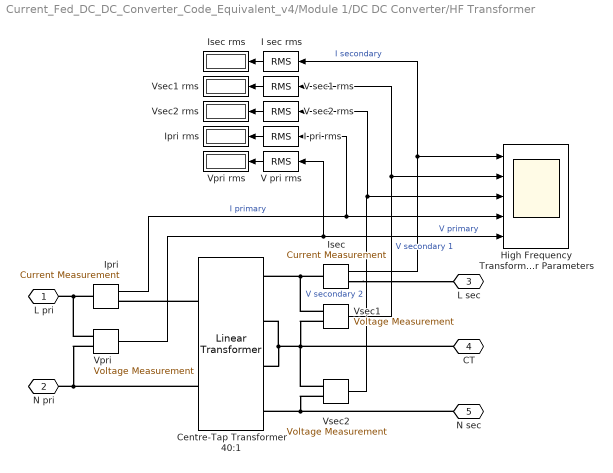
== system Current_Fed_DC_DC_Converter_Code_Equivalent_v4/Module 1/DC DC Converter/HF Transformer ==
  Centre-Tap Transformer 40:1 : powerlib/Elements/Linear Transformer  UNITS=SI  NominalPower=[P_TX f_sw]  winding1=[V_pri R_leak L_leak]  winding2=[V_sec R_leak L_leak]  ThreeWindings=on  winding3=[V_sec R_leak L_leak]  RmLm=[R_mag L_mag]  Measurements=None  DataType=on
  High Frequency Transformer Parameters : Scope  NumInputPorts=5
  I pri rms : powerlib_meascontrol/Measurements/RMS  TrueRMS=on  Freq=f_supply  RMSInit=0  Ts=0
  I sec rms : powerlib_meascontrol/Measurements/RMS  TrueRMS=on  Freq=f_supply  RMSInit=0  Ts=0
  Ipri : powerlib/Measurements/Current Measurement  PhasorSimulation=off  OutputType=Complex  PSBequivalent=0
  Ipri rms : Display
  Isec : powerlib/Measurements/Current Measurement  PhasorSimulation=off  OutputType=Complex  PSBequivalent=0
  Isec rms : Display
  V pri rms : powerlib_meascontrol/Measurements/RMS  TrueRMS=on  Freq=f_supply  RMSInit=0  Ts=0
  V sec1 rms : powerlib_meascontrol/Measurements/RMS  TrueRMS=on  Freq=f_supply  RMSInit=0  Ts=0
  V sec2 rms : powerlib_meascontrol/Measurements/RMS  TrueRMS=on  Freq=f_supply  RMSInit=0  Ts=0
  Vpri : powerlib/Measurements/Voltage Measurement  PhasorSimulation=off  OutputType=Complex  PSBequivalent=0
  Vpri rms : Display
  Vsec1 : powerlib/Measurements/Voltage Measurement  PhasorSimulation=off  OutputType=Complex  PSBequivalent=0
  Vsec1 rms : Display
  Vsec2 : powerlib/Measurements/Voltage Measurement  PhasorSimulation=off  OutputType=Complex  PSBequivalent=0
  Vsec2 rms : Display
  L pri : PMIOPort  Side=Left
  N pri : PMIOPort  Port=2  Side=Left
  L sec : PMIOPort  Port=3  Side=Right
  CT : PMIOPort  Port=4  Side=Right
  N sec : PMIOPort  Port=5  Side=Right
  wires:
  Isec/1 -> High Frequency Transformer Parameters/1, I sec rms/1  "I secondary"
  Vsec1/1 -> V sec1 rms/1, High Frequency Transformer Parameters/2  "V secondary 1"
  Vsec2/1 -> V sec2 rms/1, High Frequency Transformer Parameters/3  "V secondary 2"
  Ipri/1 -> I pri rms/1, High Frequency Transformer Parameters/4  "I primary"
  Vpri/1 -> High Frequency Transformer Parameters/5, V pri rms/1  "V primary"
  I sec rms/1 -> Isec rms/1
  V sec1 rms/1 -> Vsec1 rms/1
  V sec2 rms/1 -> Vsec2 rms/1
  V pri rms/1 -> Vpri rms/1
  I pri rms/1 -> Ipri rms/1
  connections:
  Centre-Tap Transformer 40:1/LConn2 -- Vpri/LConn2 -- N pri/RConn1
  Ipri/LConn1 -- L pri/RConn1 -- Vpri/LConn1
  CT/RConn1 -- Vsec1/LConn2 -- Vsec2/LConn1 -- Centre-Tap Transformer 40:1/RConn2 -- Centre-Tap Transformer 40:1/RConn3
  N sec/RConn1 -- Vsec2/LConn2 -- Centre-Tap Transformer 40:1/RConn4
  Centre-Tap Transformer 40:1/LConn1 -- Ipri/RConn1
  Isec/RConn1 -- L sec/RConn1
  Isec/LConn1 -- Vsec1/LConn1 -- Centre-Tap Transformer 40:1/RConn1

== system Current_Fed_DC_DC_Converter_Code_Equivalent_v4/Module 1/DC DC Converter/Inverter ==
  Iref : Inport
  Ifeed : Inport  Port=2
  Vfeed : Inport  Port=3
  Converter : Subsystem
      settings: PortSchema="{\"entries\":[{\"content\":{\"sides\":[{\"content\":{\"connectorIds\":[\"LConn1\",\"LConn2\"]},\"type\":\"ConnectorPlacement.EquallySpacedRectSide\",\"uuid\":\"0645cdc9-e655-49ab-a1d8-1293a5a1d66e\"},{\"content\":{\"connectorIds\":[\"RConn1\",\"RConn2\"],\"side\":\"RIGHT\"},\"type\":\"ConnectorPlacement.EquallySpacedRectSide\",\"uuid\":\"2ef7d2b0-2c84-4192-a188-141ae61cdfda\"},{\"content\":{\"connectorIds\":[\"In1\"],\"side\":\"TOP\"},\"type\":\"ConnectorPlacement.EquallySpacedRectSide\",\"uuid\":\"c5fd5dee-0ba9-4cec-8a2b-47382b263168\"}]},\"type\":\"ConnectorPlacement.EquallySpacedConnector\",\"uuid\":\"4d765392-2146-4c23-badc-b27487fa349e\"}],\"packageUris\":[\"http://schema.mathworks.com/mf0/Connector/19700101\"],\"version\":\"1.0\"}"
  Pulse Generator : Subsystem
  +ve : PMIOPort  Side=Left
  -ve : PMIOPort  Port=2  Side=Left
  Line : PMIOPort  Port=3  Side=Right
  Neutral : PMIOPort  Port=4  Side=Right
  Iref Main : Outport
  wires:
  Vfeed/1 -> Pulse Generator/3(V Feed)
  Pulse Generator/1(Pulses) -> Converter/1(Pulses)
  Ifeed/1 -> Pulse Generator/2(I feed)
  Pulse Generator/2(Iref Main) -> Iref Main/1
  Iref/1 -> Pulse Generator/1(Iref)
  connections:
  Converter/LConn2 -- -ve/RConn1
  Converter/LConn1 -- +ve/RConn1
  Converter/RConn1 -- Line/RConn1
  Converter/RConn2 -- Neutral/RConn1

== system Current_Fed_DC_DC_Converter_Code_Equivalent_v4/Module 1/DC DC Converter/Sensor ==
  Iin : Inport
  Vin : Inport  Port=2
  Current 12bit ADC : Gain  Gain=ADC_Res
  Current Transducer : Gain  Gain=I_sense
  Voltage 12bit ADC : Gain  Gain=ADC_Res
  Voltage Transducer : Gain  Gain=V_sense
  Iout : Outport
  Vout : Outport  Port=2
  wires:
  Iin/1 -> Current Transducer/1
  Current Transducer/1 -> Current 12bit ADC/1
  Voltage Transducer/1 -> Voltage 12bit ADC/1
  Current 12bit ADC/1 -> Iout/1
  Voltage 12bit ADC/1 -> Vout/1
  Vin/1 -> Voltage Transducer/1

== system Current_Fed_DC_DC_Converter_Code_Equivalent_v4/Module 2/3 Phase Rectifier/3 Phase Rectifier ==
  D{1..6} (6 alike) : powerlib/Power Electronics/Diode  Ron=0.001  Lon=0  Vf=0.8  IC=0  UseSnubber=0  Rs=500  Cs=250e-9  Measurements=on
  D1 V&I : Scope  Commented=on
  D2 V&I : Scope  Commented=on
  D3 V&I : Scope  Commented=on
  D4 V&I : Scope  Commented=on
  D5 V&I : Scope  Commented=on
  D6 V&I : Scope  Commented=on
  R Phase : PMIOPort  Side=Left
  Y Phase : PMIOPort  Port=2  Side=Left
  B Phase : PMIOPort  Port=3  Side=Left
  +ve : PMIOPort  Port=4  Side=Right
  -ve : PMIOPort  Port=5  Side=Right
  wires:
  D1/1 -> D1 V&I/1
  D4/1 -> D4 V&I/1
  D3/1 -> D3 V&I/1
  D5/1 -> D5 V&I/1
  D2/1 -> D2 V&I/1
  D6/1 -> D6 V&I/1
  connections:
  B Phase/RConn1 -- D2/RConn1 -- D5/LConn1
  Y Phase/RConn1 -- D4/RConn1 -- D3/LConn1
  -ve/RConn1 -- D2/LConn1 -- D4/LConn1 -- D6/LConn1
  D5/RConn1 -- +ve/RConn1 -- D3/RConn1 -- D1/RConn1
  R Phase/RConn1 -- D6/RConn1 -- D1/LConn1

== system Current_Fed_DC_DC_Converter_Code_Equivalent_v4/Module 2/3 Phase Rectifier/Filter ==
  Cdc 1 : powerlib/Elements/Series RLC Branch  LConnTagsString=__new0  RConnTagsString=__new0  BranchType=C  Resistance=1  Inductance=1e-3  SetiL0=off  InitialCurrent=0  Capacitance=2*C_filt  Setx0=off  InitialVoltage=0  Measurements=None
  Cdc 2 : powerlib/Elements/Series RLC Branch  LConnTagsString=__new0  RConnTagsString=__new0  BranchType=C  Resistance=1  Inductance=1e-3  SetiL0=off  InitialCurrent=0  Capacitance=2*C_filt  Setx0=off  InitialVoltage=0  Measurements=None
  DC Bus Filter Parameters : Scope  NumInputPorts=2
  Iout : powerlib/Measurements/Current Measurement  PhasorSimulation=off  OutputType=Complex  PSBequivalent=0
  Vout : powerlib/Measurements/Voltage Measurement  PhasorSimulation=off  OutputType=Complex  PSBequivalent=0
  +ve IN : PMIOPort  Side=Left
  -ve In : PMIOPort  Port=2  Side=Left
  +ve OUT : PMIOPort  Port=3  Side=Right
  Mid : PMIOPort  Port=4  Side=Right
  -ve OUT : PMIOPort  Port=5  Side=Right
  wires:
  Vout/1 -> DC Bus Filter Parameters/2  "Vout"
  Iout/1 -> DC Bus Filter Parameters/1  "Iout"
  connections:
  Mid/RConn1 -- Cdc 2/LConn1 -- Cdc 1/RConn1
  +ve OUT/RConn1 -- Iout/RConn1
  -ve OUT/RConn1 -- -ve In/RConn1 -- Cdc 2/RConn1 -- Vout/LConn2
  Iout/LConn1 -- +ve IN/RConn1 -- Cdc 1/LConn1 -- Vout/LConn1

== system Current_Fed_DC_DC_Converter_Code_Equivalent_v4/Module 2/DC DC Converter/Centre Tap Rectifier ==
  D1 : powerlib/Power Electronics/Diode  Ron=0.001  Lon=0  Vf=0.8  IC=0  UseSnubber=0  Rs=500  Cs=250e-9  Measurements=on
  D1 V&I : Scope  Commented=on
  D2 : powerlib/Power Electronics/Diode  Ron=0.001  Lon=0  Vf=0.8  IC=0  UseSnubber=0  Rs=500  Cs=250e-9  Measurements=on
  D2 V&I1 : Scope  Commented=on
  Line : PMIOPort  Side=Left
  Centre-tap : PMIOPort  Port=2  Side=Left
  Neutral : PMIOPort  Port=3  Side=Left
  +ve : PMIOPort  Port=4  Side=Right
  -ve : PMIOPort  Port=5  Side=Right
  wires:
  D1/1 -> D1 V&I/1
  D2/1 -> D2 V&I1/1
  connections:
  D1/RConn1 -- +ve/RConn1 -- D2/RConn1
  D1/LConn1 -- Line/RConn1
  D2/LConn1 -- Neutral/RConn1
  -ve/RConn1 -- Centre-tap/RConn1

== system Current_Fed_DC_DC_Converter_Code_Equivalent_v4/Module 2/DC DC Converter/Chopper ==
  Chop Pulse Generator : Subsystem
  Fault Detection : Subsystem
  Io avg : powerlib_meascontrol/Measurements/Mean  Freq=f_supply  Vinit=0  Ts=0
  Iout : powerlib/Measurements/Current Measurement  PhasorSimulation=off  OutputType=Complex  PSBequivalent=0
  Out Parameters : Scope  NumInputPorts=2
  Qchop : powerlib/Power Electronics/IGBT  Ron=0.001  Lon=0  Vf=1  Tf=1e-6  Tt=2e-6  IC=0  Rs=1e5  Cs=inf  Measurements=on
  Qchop V&I : Scope  Commented=on
  Rchop : powerlib/Elements/Series RLC Branch  LConnTagsString=__new0  RConnTagsString=__new0  BranchType=R  Resistance=0.1  Inductance=1e-3  SetiL0=off  InitialCurrent=0  Capacitance=1e-6  Setx0=off  InitialVoltage=0  Measurements=None
  Vo avg : powerlib_meascontrol/Measurements/Mean  Freq=f_supply  Vinit=0  Ts=0
  Vout : powerlib/Measurements/Voltage Measurement  PhasorSimulation=off  OutputType=Complex  PSBequivalent=0
  +ve IN : PMIOPort  Side=Left
  -ve IN : PMIOPort  Port=2  Side=Left
  +ve OUT : PMIOPort  Port=3  Side=Right
  -ve OUT : PMIOPort  Port=4  Side=Right
  Idc avg : Outport
  Vdc avg : Outport  Port=2
  Vdc : Outport  Port=3
  " Idc" : Outport  Port=4
  wires:
  Chop Pulse Generator/1(Chop Pulse) -> Qchop/1
  Vo avg/1 -> Vdc avg/1  "Vo avg"
  Qchop/1 -> Qchop V&I/1
  Iout/1 -> " Idc"/1, Fault Detection/2(I Output), Io avg/1, Out Parameters/1  "Iout"
  Io avg/1 -> Idc avg/1  "Io avg"
  Vout/1 -> Vdc/1, Vo avg/1, Out Parameters/2, Fault Detection/1(V Output)  "Vout"
  Fault Detection/1(OV Fault) -> Chop Pulse Generator/1(Over Voltage Fault)
  connections:
  +ve OUT/RConn1 -- Iout/RConn1 -- Vout/LConn1
  Rchop/LConn1 -- Qchop/RConn1
  Iout/LConn1 -- +ve IN/RConn1 -- Qchop/LConn1
  -ve OUT/RConn1 -- -ve IN/RConn1 -- Rchop/RConn1 -- Vout/LConn2
